simulink model "GP_FeLi"  (R2019a)
settings: Solver=FixedStepAuto  StartTime=0  StopTime=120  FixedStep=0.005  RelTol=1e-3
model workspace: external: MAT-File (data not in the file)
libraries: RealTimeLearning x2, simulink x1
settings Model: SnapshotBufferSize=1  SnapshotInterval=1  Creator=aordonez  LastModifiedBy=alederer
settings SolverCC: AlgebraicLoopSolver=LineSearch
settings DataIOCC: SaveFormat=Array
settings DebuggingCC: PregeneratedLibrarySubsystemCodeDiagnostic=none  ArithmeticOperatorsInVariantConditions=warning
settings CodeAppCC: StateflowObjectComments=on

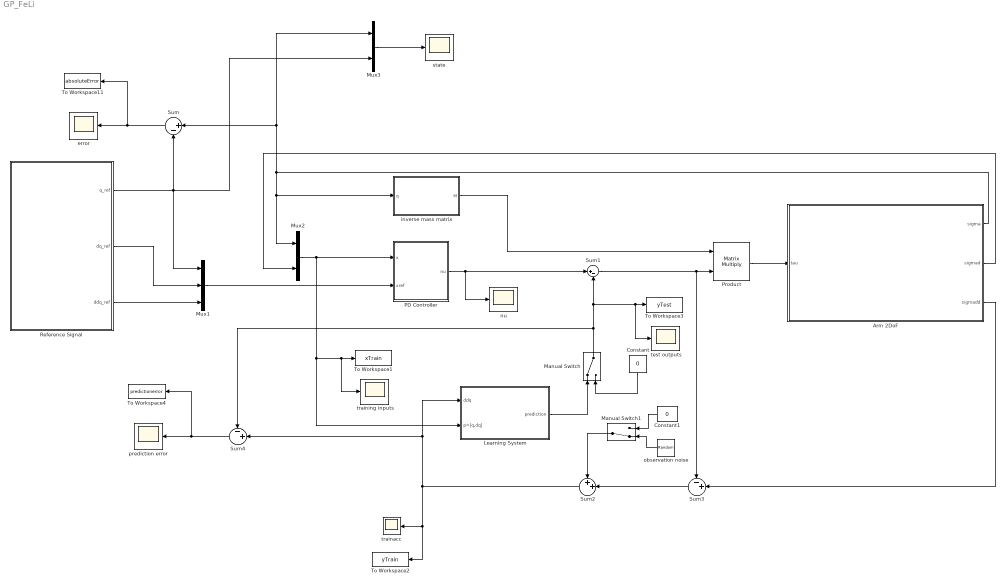
== system GP_FeLi ==
  Arm 2DoF : Subsystem
  Constant : Constant  Value=0
  Constant1 : Constant  Value=0
  Learning System : Subsystem
  Manual Switch : ManualSwitch
  Manual Switch1 : ManualSwitch  CurrentSetting=0
  Mux1 : Mux  Inputs=3
  Mux2 : Mux  Inputs=2
  Mux3 : Mux  Inputs=2
  PD Controller : MATLAB Function  TreatAsAtomicUnit=on
  Product : Product  Multiplication=Matrix(*)
  Reference Signal : Subsystem
  Sum : Sum  Inputs=|+-
  Sum1 : Sum  Inputs=|+-
  Sum2 : Sum  Inputs=++|
  Sum3 : Sum  Inputs=-+|
  Sum4 : Sum  Inputs=-+|
  To Workspace1 : ToWorkspace  VariableName=xTrain  SampleTime=-1
      settings: Save2DSignal=2-D array (concatenate along first dimension)
  To Workspace11 : ToWorkspace  VariableName=absoluteError  SampleTime=-1
      settings: Save2DSignal=2-D array (concatenate along first dimension)
  To Workspace2 : ToWorkspace  VariableName=yTrain  SampleTime=-1
      settings: Save2DSignal=2-D array (concatenate along first dimension)
  To Workspace3 : ToWorkspace  VariableName=yTest  SampleTime=-1
      settings: Save2DSignal=2-D array (concatenate along first dimension)
  To Workspace4 : ToWorkspace  VariableName=predictionerror  SampleTime=-1
      settings: Save2DSignal=2-D array (concatenate along first dimension)
  error : Scope
  inverse mass matrix : MATLAB Function  TreatAsAtomicUnit=on
  nu : Scope
  observation noise : RandomNumber  SampleTime=0.005
  prediction error : Scope
  state : Scope
  test outputs : Scope
  trainacc : Scope
  training inputs : Scope
  wires:
  Arm 2DoF/2(sigmad) -> Mux2/2
  Sum/1 -> To Workspace11/1, error/1
  Mux2/1 -> PD Controller/1(x), training inputs/1, To Workspace1/1, Learning System/2(p=[q,dq])
  Constant/1 -> Manual Switch/2
  Reference Signal/3(ddq_ref) -> Mux1/3
  Constant1/1 -> Manual Switch1/1
  observation noise/1 -> Manual Switch1/2
  Mux1/1 -> PD Controller/2(xref)
  Reference Signal/2(dq_ref) -> Mux1/2
  Reference Signal/1(q_ref) -> Mux3/2, Mux1/1, Sum/2
  Arm 2DoF/1(sigma) -> Mux3/1, Sum/1, Mux2/1, inverse mass matrix/1(q)
  inverse mass matrix/1(M) -> Product/1
  Sum1/1 -> Product/2, Sum3/1
  Manual Switch1/1 -> Sum2/1
  Learning System/1(prediction) -> Manual Switch/1
  Mux3/1 -> state/1
  Sum3/1 -> Sum2/2
  PD Controller/1(nu) -> nu/1, Sum1/1
  Arm 2DoF/3(sigmadd) -> Sum3/2
  Sum4/1 -> To Workspace4/1, prediction error/1
  Manual Switch/1 -> Sum4/1, test outputs/1, To Workspace3/1, Sum1/2
  Sum2/1 -> Learning System/1(ddq), Sum4/2, To Workspace2/1, trainacc/1
  Product/1 -> Arm 2DoF/1(tau)

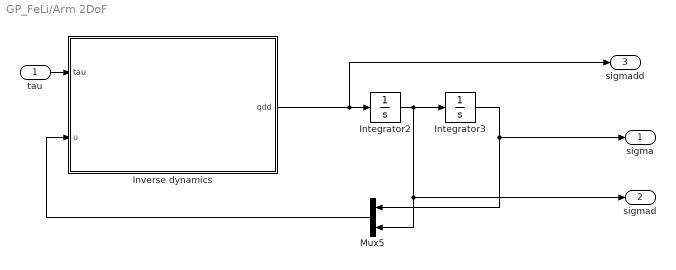
== system GP_FeLi/Arm 2DoF ==
  tau : Inport
  Integrator2 : Integrator  InitialCondition=[0;0]
  Integrator3 : Integrator  InitialCondition=[0;0]
  Inverse dynamics : MATLAB Function  TreatAsAtomicUnit=on
  Mux5 : Mux  Inputs=2
  sigma : Outport
  sigmad : Outport  Port=2
  sigmadd : Outport  Port=3
  wires:
  Integrator3/1 -> sigma/1, Mux5/1
  tau/1 -> Inverse dynamics/1(tau)
  Integrator2/1 -> sigmad/1, Mux5/2, Integrator3/1
  Mux5/1 -> Inverse dynamics/2(u)
  Inverse dynamics/1(qdd) -> Integrator2/1, sigmadd/1

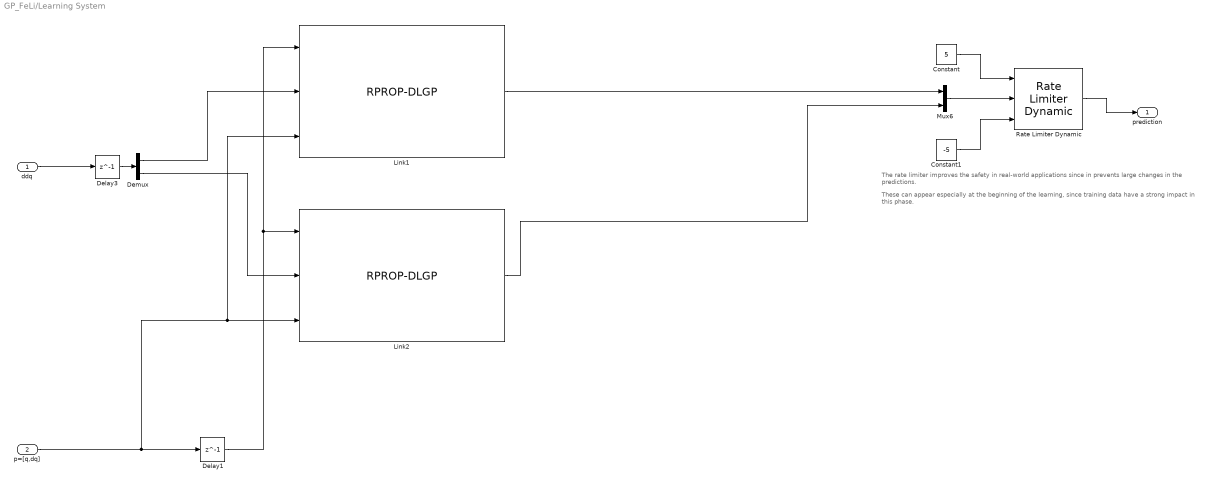
== system GP_FeLi/Learning System ==
  note: The rate limiter improves the safety in real-world applications since in prevents large changes in the predictions.
  note: These can appear especially at the beginning of the learning, since training data have a strong impact in this phase.
  ddq : Inport
  p=[q,dq] : Inport  Port=2
  Constant : Constant  Value=5
  Constant1 : Constant  Value=-5
  Delay1 : Delay  DelayLength=1
  Delay3 : Delay  DelayLength=1
  Demux : Demux  Outputs=2
  Link1 : RealTimeLearning/RPROP-DLGP  ard=on  pts=50  N=10000  xSize=4  timeRate=0.005  divMethod=3  wo=300
      settings: SourceProductName=Real Time Learning
  Link2 : RealTimeLearning/RPROP-DLGP  ard=on  pts=50  N=10000  xSize=4  timeRate=0.005  divMethod=3  wo=300
      settings: SourceProductName=Real Time Learning
  Mux6 : Mux  Inputs=2
  Rate Limiter Dynamic : simulink/Discontinuities/Rate Limiter Dynamic
      settings: SourceProductName=Simulink
  prediction : Outport
  wires:
  Delay3/1 -> Demux/1
  ddq/1 -> Delay3/1
  Demux/1 -> Link1/2
  p=[q,dq]/1 -> Link1/3, Link2/3, Delay1/1
  Delay1/1 -> Link2/1, Link1/1
  Link2/1 -> Mux6/2
  Demux/2 -> Link2/2
  Link1/1 -> Mux6/1
  Constant/1 -> Rate Limiter Dynamic/1
  Constant1/1 -> Rate Limiter Dynamic/3
  Mux6/1 -> Rate Limiter Dynamic/2
  Rate Limiter Dynamic/1 -> prediction/1

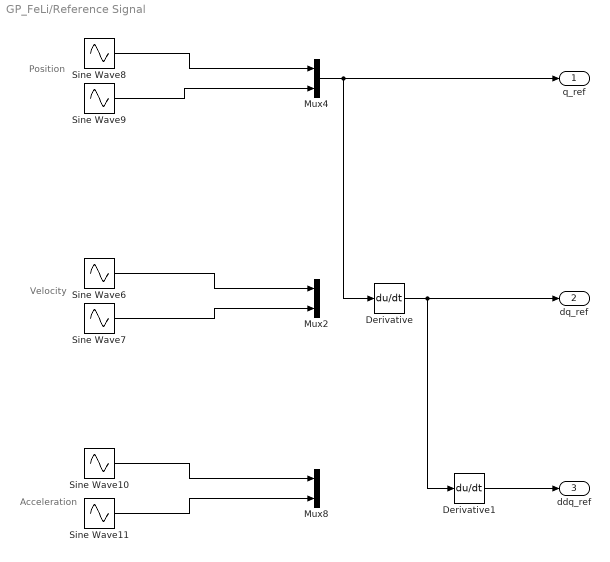
== system GP_FeLi/Reference Signal ==
  note: Velocity
  note: Position
  note: Acceleration
  Derivative : Derivative
  Derivative1 : Derivative
  Mux2 : Mux  Inputs=2
  Mux4 : Mux  Inputs=2
  Mux8 : Mux  Inputs=2
  Sine Wave10 : Sin  Amplitude=-pi/6  Phase=pi/2  SampleTime=0
  Sine Wave11 : Sin  Amplitude=-pi/24  Frequency=0.5  Phase=pi/2  SampleTime=0
  Sine Wave6 : Sin  Amplitude=-pi/6  SampleTime=0
  Sine Wave7 : Sin  Amplitude=-pi/12  Frequency=0.5  SampleTime=0
  Sine Wave8 : Sin  Amplitude=pi/6  Phase=pi/2  SampleTime=0
  Sine Wave9 : Sin  Amplitude=pi/6  Frequency=0.5  Phase=pi/2  SampleTime=0
  q_ref : Outport
  dq_ref : Outport  Port=2
  ddq_ref : Outport  Port=3
  wires:
  Sine Wave10/1 -> Mux8/1
  Mux4/1 -> Derivative/1, q_ref/1
  Sine Wave8/1 -> Mux4/1
  Sine Wave11/1 -> Mux8/2
  Sine Wave6/1 -> Mux2/1
  Sine Wave9/1 -> Mux4/2
  Sine Wave7/1 -> Mux2/2
  Derivative/1 -> Derivative1/1, dq_ref/1
  Derivative1/1 -> ddq_ref/1

== matlab function GP_FeLi/inverse mass matrix ==
  data: q input; M output
function M = fcn(q)

Iz1 = 2;   %moment of inertia
Iz2 =2;    
m1 = 2;    %mass
m2 = 2;
l1 = 2;    %length
l2 = 2;
r1 = 2;   %length to the center of mass
r2 = 2;
g = 9.81;  %gravity

a = Iz1 + Iz2 + m1*r1^2 + m2*( l1^2 + r2^2 );
b = m2*l1*r2;
d = Iz2 + m2*r2^2;

M = [ a + 2*b*cos( q(2) ),   d + b*cos( q(2) );
          d + b*cos( q(2) ),              d        ];

== matlab function GP_FeLi/PD Controller ==
  data: x input; nu output; xref input
function nu = fcn(x,xref)

nDof = size(x,1)/2;
nu = zeros(2,1);

lam=1*ones(nDof,1);
kc=2*ones(nDof,1);

e=x-xref(1:end-nDof);
nu=zeros(nDof,1);

for i=1:nDof
    mask=linspace(i,size(x,1)-2+i,nDof);
    r=[lam(i),1]*e(mask);
    nu(i)=-kc(i)*r-lam(i)*e(mask(2))+xref(end-nDof+i);
end

== matlab function GP_FeLi/Arm 2DoF/Inverse dynamics ==
  data: tau input; u input; qdd output
function qdd = fcn(tau,u)
%{
inverse dynamics of a 2 DoF robotic arm
Inputs tau: 2x1 vector. Torques
       u: 4x1 vector [sigma1, sigma2, sigma1d, sigma2d]' position and speed
Output qdd: 2x1 vector with accelerations 
%}

Iz1 = 2;   %moment of inertia
Iz2 =2;    
m1 = 2;    %mass
m2 = 2;
l1 = 2;    %length
l2 = 2;
r1 = 2;   %length to the center of mass
r2 = 2;
g = 9.81;  %gravity

a = Iz1 + Iz2 + m1*r1^2 + m2*( l1^2 + r2^2 );
b = m2*l1*r2;
d = Iz2 + m2*r2^2;

M_inv = [ a + 2*b*cos( u(2) ),   d + b*cos( u(2) );
          d + b*cos( u(2) ),              d        ]^-1;

C = [ -b*sin( u(2) )*(2*u(3)*u(4) + u(4)^2); 
            b*sin( u(2) )*u(3)^2           ];
        

N = [ m1*g*r1*cos( u(1) ) + m2*g*( l1*cos( u(1) ) + r2*cos( u(1)+u(2) ) );
                    m2*g*r2*cos( u(1)+u(2) )                              ];

qdd = M_inv*( -C - N  + tau );
